simulink model "ae2e3"  (R2022a)
settings: Solver=VariableStepAuto  StartTime=0.0  StopTime=inf  RelTol=1e-3
settings Model: Creator=attit  LastModifiedBy=attit
settings ConfigComp: DVMaxProcessTime=4000  DVModelCoverageObjectives=MCDC  DVTestSuiteOptimization=Auto  DVDetectOutOfBounds=on  DVModelReferenceHarness=on  DVHarnessSource=Signal Editor

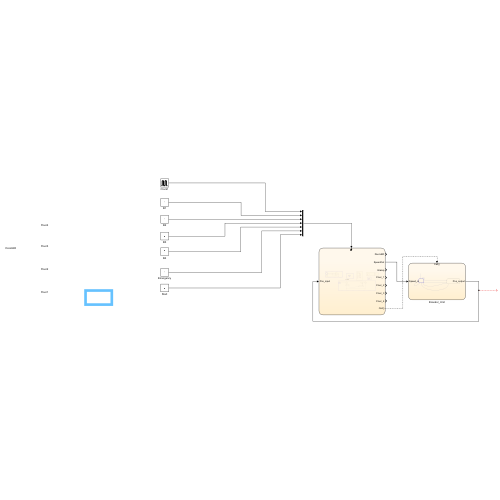
[thumbnail: Simulink's stored preview of the top-level diagram]
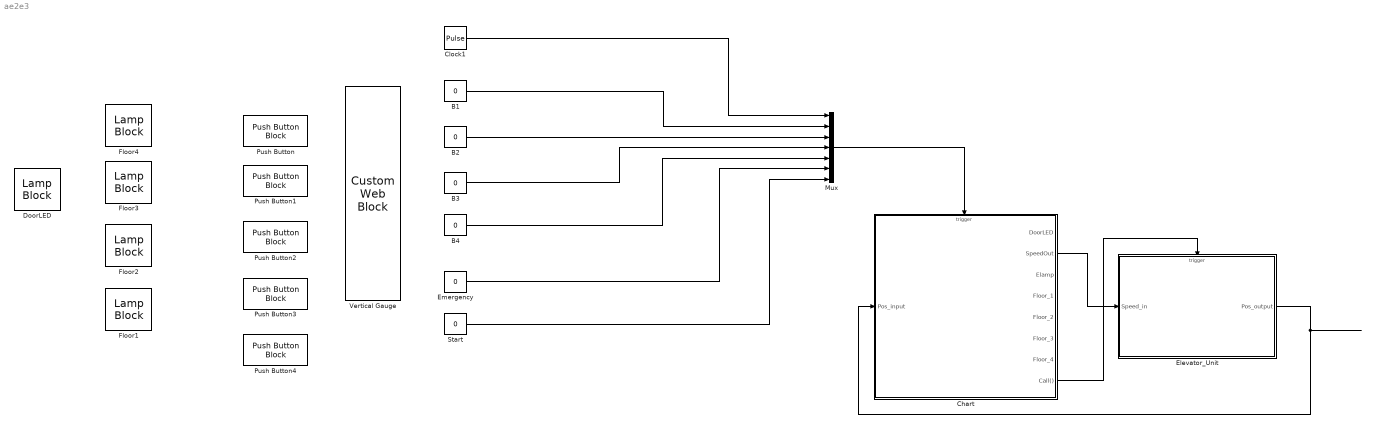
== system ae2e3 ==
  B{1..4} (4 alike) : Constant  Value=0
  Chart : Stateflow chart  TreatAsAtomicUnit=on
  Clock1 : DiscretePulseGenerator  PulseType=Time based  Period=1  PulseWidth=50
  DoorLED : LampBlock  LabelPosition=Hide
  Elevator_Unit : Stateflow chart  TreatAsAtomicUnit=on
  Emergency : Constant  Value=0
  Floor{1..4} (4 alike) : LampBlock  LabelPosition=Hide
  Mux : Mux  Inputs=7
  Push Button : PushButtonBlock  ButtonText=F4  OffValue=0.000000
  Push Button1 : PushButtonBlock  ButtonText=F3  OffValue=0.000000
  Push Button2 : PushButtonBlock  ButtonText=F2  OffValue=0.000000
  Push Button3 : PushButtonBlock  ButtonText=F1  OffValue=0.000000
  Push Button4 : PushButtonBlock  ButtonText=Emergency  OffValue=0.000000
  Start : Constant  Value=0
  Vertical Gauge : CustomWebBlock  LabelPosition=Hide  ShowInitialText=on  Configuration="{\"type\":\"LinearGauge\",\"settings\":{\"BindingType\":\"signal\",\"backgroundColor\":[0,0,0,\"1\"],\"backgroundOffset\":0,\"backgroundOpacity\":1,\"fixedAspectRatio\":\"on\",\"orientation\":\"vertical\",\"showBackgroundColor\":false,\"value\":0},\"components\":[{\"name\":\"LinearScaleComponent\",\"settings\":{\"bounds\":{\"max\":4,\"min\":1,\"tickInterval\":1},\"internalTickHeightScaleFactor\":0.5,\"labelColor\":[255,255,200],\"labelFont\":{\"font\":\"Arial\",\"fontSize\":12},\"labelTransparency\":1,\"needleImage\":{\"size\":[21,75],\"src\":\"data:image/svg+xml;base64,PHN2ZyB4bWxucz0iaHR0cDovL3d3dy53My5vcmcvMjAwMC9zdmciIHhtbG5zOnhsaW5rPSJodHRwOi8vd3d3LnczLm9yZy8xOTk5L3hsaW5rIiB2aWV3Qm94PSIwIDAgMjEgNzUiPjxkZWZzPjxzdHlsZT4uY2xzLTF7ZmlsbDpub25lO30uY2xzLTJ7aXNvbGF0aW9uOmlzb2xhdGU7fS5jbHMtM3tjbGlwLXBhdGg6dXJsKCNjbGlwLXBhdGgpO30uY2xzLTR7b3BhY2l0eTowLjM7bWl4LWJsZW5kLW1vZGU6bXVsdGlwbHk7fS5jbHMtNXtmaWxsOiNlYjI2Mjk7fTwvc3R5bGU+PGNsaXBQYXRoIGlkPSJjbGlwLXBhdGgiIHRyYW5zZm9y ...(+1928 chars)\",\"srcOrientation\":\"horizontal\"},\"needleOffset\":[0.007413509060955519,0],\"needleSize\":{\"height\":0.11955094537815127,\"width\":0.7589285714285714},\"position\":[0.015821953781512604,0.06969246031746032,0.7998511904761905,0.9641544117647058],\"referencePoint\":\"auto\",\"scaleColors\":[],\"scaleColorsSize\":0.2,\"scaleDirection\":\"BT\",\"showLabels\":1,\"showMinorTicks\":0,\"showSpanLine\":1,\"showTicks\":1,\"tickColor\":[252,252,197],\"tickTransparency\":1,\"valueBarColor\":[23,89,176],\"valueBarOffset\":0,\"valueBarSize\":0.23,\"valueBarTransparency\":1}},{\"name\":\"BackgroundImageComponent\",\"settings\":{\"image\":{\"size\":[380,101],\"src\":\"data:image/svg+xml;base64,PHN2ZyBpZD0iZnJhbWUiIHhtbG5zPSJodHRwOi8vd3d3LnczLm9yZy8yMDAwL3N2ZyIgeG1sbnM6eGxpbms9Imh0dHA6Ly93d3cudzMub3JnLzE5OTkveGxpbmsiIHZpZXdCb3g9IjAgMCAzODAgMTAxIj48ZGVmcz48c3R5bGU+LmNscy0xe2ZpbGw6IzAwMmI0Mjt9LmNscy0ye2ZpbGw6IzQyNzA4Mjt9LmNscy0ze2ZpbGw6dXJsKCNyYWRpYWwtZ3JhZGllbnQpO308L3N0eWxlPjxyYWRpYWxHcmFkaWVudCBpZD0icmFkaWFsLWdyYWRpZW50IiBjeD0iMTkwIiBjeT0iNTAuNSIgcj0iMjY5LjIxIiBncmFkaWVudFVuaXRzPSJ1c2VyU3BhY2VPblVzZSI+PHN0b3Agb2Zmc2V0PSIwLjAxIiBzdG9wLWNvbG9yPSIjM2U0ZjU4Ii8+PHN0b3Agb2Zmc2V0PSIwLjA2IiBzdG9wLWNvbG9yPSIjNDQ1NzYxIi8+PHN0b3Agb2Zmc2V0PSIwLjE1IiBzdG9wLWNvbG9yPSIjNTU2YTc2Ii8+PHN0b3Agb2Zmc2V0PSIwLjI1IiBzdG9wLWNvbG9yPSIjNmQ4ODk1Ii8+PHN0b3Agb2Zmc2V0PSIwLjM4IiBzdG9wLWNvbG9yPSIjOGZiMmMzIi8+PHN0b3Agb2Zmc2V0PSIwLjUyIiBzdG9wLWNvbG9yPSIjYjZlNGZhIi8+PHN0b3Agb2Zmc2V0PSIxIiBzdG9wLWNvbG9yPSIjMTU0NjU3Ii8+PC9yYWRpYWxHcmFkaWVudD48L2RlZnM+PGcgaWQ9IkxheWVyXzIiIGRhdGEtbmFtZT0iTGF5ZXIgMiI+PGcgaWQ9IkxheWVyXzEtMiIgZGF0YS1uYW1lPSJMYXllciAxLTIiPjxyZWN0IGlkPSJyZWN0MTAzNiIgY2xhc3M9ImNscy0xIiB4PSIxMSIgeT0iMTEiIHdpZHRoPSIzNTgiIGhlaWdodD0iNzkiLz48cGF0aCBpZD0icGF0aDEwMzgiIGNsYXNzPSJjbHMtMiIgZD0iTTgsOFY5M0gzNzJWOFpNMzY5LDkwSDExVjExSDM2OVoiLz48cGF0aCBpZD0icGF0aDEwNDAiIGNsYXNzPSJjbHMtMyIgZD0iTTAsMFYxMDFIMzgwVjBaTTM3Miw5M0g4VjhIMzcyWiIvPjwvZz48L2c+PC9zdmc+\",\"srcOrientation\":\"horizontal\"},\"position\":[0,0,1,1],\"scaleMode\":\"0\"}},{\"name\":\"ForegroundImageComponent\",\"settings\":{\"image\":{\"size\":[0,0],\"src\":\"default\",\"srcOrientation\":[]},\"isForeground\":1,\"position\":[0,0,1,1],\"scaleMode\":\"0\"}}]}"
  wires:
  B1/1 -> Mux/2
  Chart/2(SpeedOut) -> Elevator_Unit/1(Speed_in)
  Elevator_Unit/1(Pos_output) -> Chart/1(Pos_input)
  Clock1/1 -> Mux/1
  Chart/8(Call()) -> Elevator_Unit/Trigger
  Emergency/1 -> Mux/6
  B2/1 -> Mux/3
  B4/1 -> Mux/5
  Start/1 -> Mux/7
  Mux/1 -> Chart/Trigger
  B3/1 -> Mux/4

== stateflow chart ae2e3/Elevator_Unit ==
  state OFF
  state RUNNING
    during:
    Pos_output=Pos_output+Speed_in
  (default) -> OFF : {Pos_output=1}
  OFF -> OFF [order 3] : [Pos_output>4]{Pos_output=4}
  OFF -> RUNNING [order 1] : [Speed_in~=0]
  OFF -> OFF [order 2] : [Pos_output<1]{Pos_output=1}
  RUNNING -> OFF [order 3] : [Speed_in==0]
  RUNNING -> OFF [order 2] : [Speed_in<0&&Pos_output<=1]
  RUNNING -> OFF [order 1] : [Speed_in>0&&Pos_output>=4]
  data: Speed_in input; Pos_output output
  events: Call input FUNCTION_CALL_EVENT

== stateflow chart ae2e3/Chart ==
  state ElevatorUnitControl [parallel]
    settings: executionOrder=4
    state GO_DOWN
      entry:
      SpeedOut=-0.2
    state OFF
      entry:SpeedOut=0;
      Elamp=0;
    state GO_UP
      entry:SpeedOut=0.2
    state HALT
      entry:SpeedOut=0;
      Elamp=1
    (default) -> OFF
    OFF -> (junction 166) [order 1] : [in(LiftAlgorithm.MOTOR_ON)]
    (junction 166) -> GO_DOWN [order 1] : [Direction<Pos_input]
    GO_DOWN -> (junction 182) [order 1] : [Emergency]
    (junction 166) -> (junction 177) [order 2] : [Direction>Pos_input]
    (junction 182) -> (junction 183)
    GO_DOWN -> OFF [order 2] : [~in(LiftAlgorithm.MOTOR_ON)]
    GO_UP -> OFF [order 2] : [~in(LiftAlgorithm.MOTOR_ON)]
    HALT -> OFF : [Start]
    OFF -> HALT [order 2] : [Emergency]
    (junction 177) -> GO_UP
    GO_UP -> (junction 183) [order 1] : [Emergency]
    (junction 183) -> (junction 184)
    (junction 184) -> HALT
  state RequestServiced(pos) [function]
    note: Do not put any code along
        | the transitions that run
        | down the right side!
    (default) -> (junction 121)
    (junction 121) -> (junction 116) [order 1] : [pos == 1]
    (junction 121) -> (junction 131) [order 2]
    (junction 116) -> (junction 137) : {F1_press=0;}
    (junction 137) -> (junction 120)
    (junction 120) -> (junction 117)
    (junction 131) -> (junction 113) [order 1] : [pos == 2]
    (junction 131) -> (junction 123) [order 2]
    (junction 113) -> (junction 135) : {F2_press=0;}
    (junction 135) -> (junction 117)
    (junction 117) -> (junction 114)
    (junction 123) -> (junction 136) [order 1] : [pos == 3]
    (junction 123) -> (junction 122) [order 2]
    (junction 136) -> (junction 118) : {F3_press=0;}
    (junction 118) -> (junction 114)
    (junction 114) -> (junction 124)
    (junction 122) -> (junction 119) [order 1] : [pos == 4]
    (junction 122) -> (junction 125) [order 2]
    (junction 119) -> (junction 115) : {F4_press=0;}
    (junction 115) -> (junction 124)
    (junction 124) -> (junction 127)
    (junction 127) -> (junction 125)
    (junction 125) -> (junction 129)
  state ret =ValidFloor(indx) [function]
    (default) -> (junction 104)
    (junction 104) -> (junction 110) [order 1] : [abs(indx-1.0)<0.1||abs(indx-2.0)<0.1||abs(indx-3.0)<0.1||abs(indx-4.0)<0.1]
    (junction 110) -> (junction 106) : {ret=1}
    (junction 104) -> (junction 106) [order 2] : {ret=0}
    (junction 106) -> (junction 103)
  state Add(Floor) [function]
    (default) -> (junction 29) : {PressCount=PressCount+1;}
    (junction 29) -> (junction 31) : {Queue(PressCount)=Floor}
  state FloorRequestProcess [parallel]
    settings: executionOrder=1
    state RequestWait
    RequestWait -> RequestWait [order 1] : [F1_evt&&Floor_1~=1]{Add(1);Floor_1=1}
    RequestWait -> RequestWait [order 4] : [F4_evt&&Floor_4~=1]{Add(4);Floor_4=1}
    RequestWait -> RequestWait [order 3] : [F3_evt&&Floor_3~=1]{Add(3);Floor_3=1}
    RequestWait -> RequestWait [order 2] : [F2_evt&&Floor_2~=1]{Add(2);Floor_2=1}
  state Trigger [parallel]
    settings: executionOrder=2
    state TriggerNextchart
    (default) -> TriggerNextchart
    TriggerNextchart -> TriggerNextchart : {Call}
  note: LIFT_ALGORITHM
  state LiftAlgorithm [parallel]
    settings: executionOrder=3
    state DOOR_WAIT
      entry:DoorLED=1;
      RequestServiced(round(Pos_input));
    state DOOR_DONE
      entry:DoorLED=0;
    state WAIT
    state REQUEST_ACCEPTED
    state MOTOR_ON
    state REQUESTED_FLOOR_FOUND
      entry:PressCount=PressCount-1;
      Queue=[Queue(Queue~=round(Pos_input)) zeros(1,length(Queue)-length(Queue(Queue~=round(Pos_input))))];
    (junction 76) -> (junction 75)
    (junction 82) -> (junction 76)
    (default) -> WAIT : {Floor_1=0;Floor_2=0;Floor_3=0;Floor_4=0; Queue=[0 0 0 0]; PressCount=0;}
    (junction 75) -> WAIT
    DOOR_DONE -> (junction 82) [order 2] : [Direction==0]
    DOOR_WAIT -> DOOR_DONE : [after(5,sec)]
    WAIT -> REQUEST_ACCEPTED : [PressCount>0]{Direction=Queue(1)}
    REQUEST_ACCEPTED -> DOOR_WAIT [order 2] : [Direction==Pos_input]{Direction=0;Queue=[Queue(Queue~=round(Pos_input)) zeros(1,length(Queue)-length(Queue(Queue~=round(Pos_input))))];}
    REQUESTED_FLOOR_FOUND -> DOOR_WAIT [order 2]
    REQUESTED_FLOOR_FOUND -> DOOR_WAIT [order 1] : [abs(Direction-Pos_input)<0.1]{Direction=0;}
    DOOR_DONE -> (junction 78) [order 1] : [Direction~=0]
    REQUEST_ACCEPTED -> MOTOR_ON [order 1] : [Direction~=Pos_input]
    (junction 79) -> MOTOR_ON
    MOTOR_ON -> REQUESTED_FLOOR_FOUND : [1==ValidFloor(Pos_input)&&1==any(Queue(:)==round(Pos_input))]
    (junction 78) -> (junction 79)
  note: ElevatorUnitControl
  (default) -> RequestWait : {Floor_1=0;Floor_2=0;Floor_3=0;Floor_4=0; Queue=[0 0 0 0]; PressCount=0;}
  data: pos function_input; indx function_input; ret function_output; Floor function_input; Queue local size=[1 4]; Pos_input input [1..4]; DoorLED output; PressCount local; Direction local; SpeedOut output; Elamp output; Floor_1 output; Floor_2 output; Floor_3 output; Floor_4 output
  events: Trigger input RISING_EDGE_EVENT; Call output FUNCTION_CALL_EVENT; F1_evt input RISING_EDGE_EVENT; F2_evt input RISING_EDGE_EVENT; F3_evt input RISING_EDGE_EVENT; F4_evt input RISING_EDGE_EVENT; Start input RISING_EDGE_EVENT; Emergency input RISING_EDGE_EVENT
